simulink model "subsysChanged"  (R2023b)
settings: Solver=VariableStepAuto  StartTime=0.0  StopTime=10.0  RelTol=1e-3
settings Model: Creator=neham  LastModifiedBy=neham

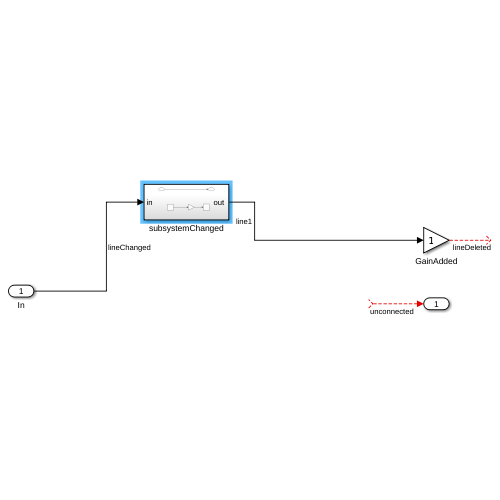
[thumbnail: Simulink's stored preview of the top-level diagram]
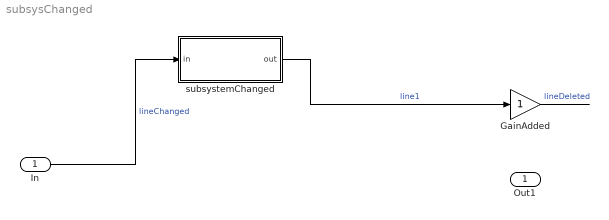
== system subsysChanged ==
  In : Inport
  GainAdded : Gain
  subsystemChanged : Subsystem
  Out1 : Outport
  wires:
  subsystemChanged/1("out ") -> GainAdded/1  "line1"
  In/1 -> subsystemChanged/1("in ")  "lineChanged"
  GainAdded/1 -> ?  "lineDeleted"
  ? -> Out1/1  "unconnected"

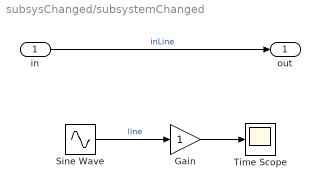
== system subsysChanged/subsystemChanged ==
  "in " : Inport
  Gain : Gain
  Sine Wave : Sin  SampleTime=0
  Time Scope : Scope
  "out " : Outport
  wires:
  "in "/1 -> "out "/1  "inLine"
  Sine Wave/1 -> Gain/1  "line"
  Gain/1 -> Time Scope/1
